simulink model "lateral_longiitude_distance"  (R2018a)
settings: Solver=FixedStepDiscrete  StartTime=0.0  StopTime=10.0  FixedStep=1  RelTol=1e-3
undefined symbols (not defined in the file or in its folder): BRAKING_ON_OFF, MUST_REQ
libraries: simulink x27
settings Model: Creator=S M Engineers  LastModifiedBy=S M Engineers

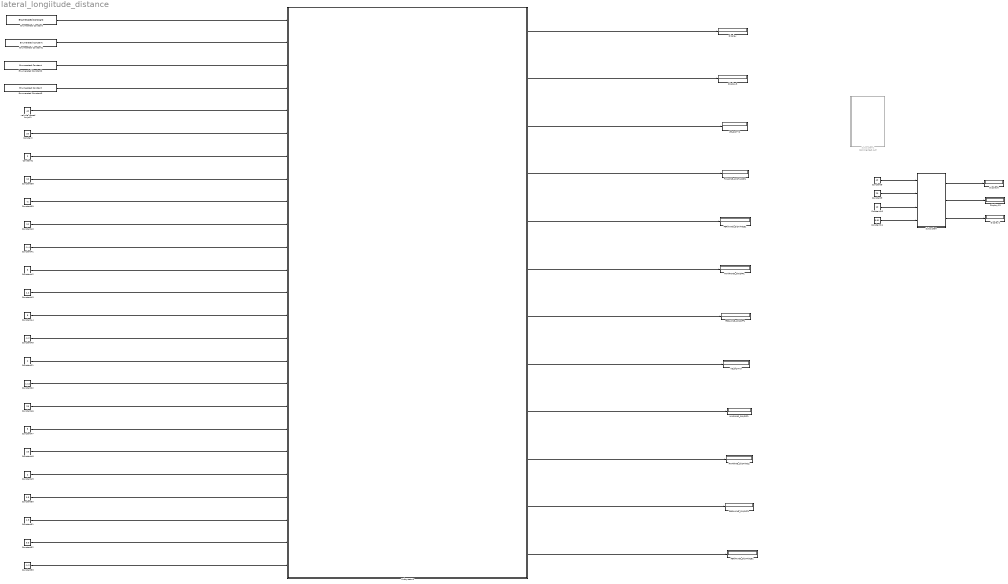
== system lateral_longiitude_distance ==
  Constant : Constant  Value=20
  Constant1 : Constant  Value=2
  Constant10 : Constant  Value=10
  Constant11 : Constant  Value=9.81
  Constant21 : Constant  Value=2
  Constant22 : Constant  Value=1.12
  Constant38 : Constant  Value=10
  Constant39 : Constant  Value=-2
  Constant40 : Constant  Value=12
  Constant41 : Constant  Value=-1.4
  Constant42 : Constant  Value=5
  Constant43 : Constant  Value=1.2
  Constant44 : Constant  Value=8
  Constant45 : Constant  Value=-1.2
  Constant46 : Constant  Value=25
  Constant47 : Constant  Value=5
  Constant48 : Constant  Value=16
  Constant49 : Constant  Value=2
  Constant50 : Constant  Value=0.5
  Constant51 : Constant  Value=1.3
  Constant52 : Constant  Value=0.3
  Constant53 : Constant  Value=-1.2
  Constant8 : Constant  Value=40
  Constant9 : Constant  Value=20
  Display{,2..3,6,13} (5 alike) : Display
  Enumerated Constant : simulink/Sources/Enumerated Constant  OutDataTypeStr=Enum: MUST_REQ  Value=MUST_REQ.IGNITION_ON  SampleTime=inf
      settings: SourceProductName=Simulink
  Enumerated Constant1 : simulink/Sources/Enumerated Constant  OutDataTypeStr=Enum: MUST_REQ  Value=MUST_REQ.EMERGENCY_BRAKING_ON  SampleTime=inf
      settings: SourceProductName=Simulink
  Enumerated Constant2 : simulink/Sources/Enumerated Constant  OutDataTypeStr=Enum: MUST_REQ  Value=MUST_REQ.DRIVE_MODE_ON  SampleTime=inf
      settings: SourceProductName=Simulink
  Enumerated Constant3 : simulink/Sources/Enumerated Constant  OutDataTypeStr=Enum: MUST_REQ  Value=MUST_REQ.REAR_MODE_OFF  SampleTime=inf
      settings: SourceProductName=Simulink
  FBRAIKNG_ON/OFF1 : Display
  FBRAKING_DISTANCE1 : Display
  FWARING_DISTANCE1 : Display
  FWARNING_ON/OFF1 : Display
  RBRAIKNG_ON/OFF1 : Display
  RBRAKING_DISTANCE1 : Display
  RWARING_DISTANC2 : Display
  Subsystem : Subsystem
  Subsystem1 : Subsystem  Commented=on
  Subsystem3 : Subsystem
      mask Display: image('Autonomous-Emergency-Braking-System-Market.jpg');
  VELOCITY2 : Display
  VELOCITY3 : Display
  WARNING_ON/OFF1 : Display
  vehicle speed km/ph1 : Constant  Value=40
  wires:
  Constant8/1 -> Subsystem/1(In1)
  Constant9/1 -> Subsystem/2(In2)
  Constant10/1 -> Subsystem/3(In3)
  Constant11/1 -> Subsystem/4(In4)
  Subsystem/1(Out1) -> Display6/1
  Subsystem/2(Out2) -> Display13/1
  Subsystem/3(Out3) -> Display2/1
  Enumerated Constant/1 -> Subsystem3/1(In1)
  Enumerated Constant1/1 -> Subsystem3/2(In2)
  Enumerated Constant2/1 -> Subsystem3/3(In3)
  Enumerated Constant3/1 -> Subsystem3/4(In4)
  vehicle speed km/ph1/1 -> Subsystem3/5(In5)
  Constant/1 -> Subsystem3/6(In6)
  Constant1/1 -> Subsystem3/7(In7)
  Constant38/1 -> Subsystem3/8(In8)
  Constant39/1 -> Subsystem3/9(In9)
  Constant40/1 -> Subsystem3/10(In10)
  Constant41/1 -> Subsystem3/11(In11)
  Constant42/1 -> Subsystem3/12(In12)
  Constant43/1 -> Subsystem3/13(In13)
  Constant44/1 -> Subsystem3/14(In14)
  Constant45/1 -> Subsystem3/15(In15)
  Constant21/1 -> Subsystem3/16(In16)
  Constant22/1 -> Subsystem3/17(In17)
  Constant46/1 -> Subsystem3/18(In18)
  Constant47/1 -> Subsystem3/19(In19)
  Constant48/1 -> Subsystem3/20(In20)
  Constant49/1 -> Subsystem3/21(In21)
  Constant50/1 -> Subsystem3/22(In22)
  Constant51/1 -> Subsystem3/23(In23)
  Constant52/1 -> Subsystem3/24(In24)
  Constant53/1 -> Subsystem3/25(In25)
  Subsystem3/1(Out1) -> Display/1
  Subsystem3/2(Out2) -> Display3/1
  Subsystem3/3(Out3) -> VELOCITY2/1
  Subsystem3/4(Out4) -> FWARING_DISTANCE1/1
  Subsystem3/5(Out5) -> FBRAKING_DISTANCE1/1
  Subsystem3/6(Out6) -> FWARNING_ON/OFF1/1
  Subsystem3/7(Out7) -> FBRAIKNG_ON/OFF1/1
  Subsystem3/8(Out8) -> VELOCITY3/1
  Subsystem3/9(Out9) -> WARNING_ON/OFF1/1
  Subsystem3/10(Out10) -> RWARING_DISTANC2/1
  Subsystem3/11(Out11) -> RBRAIKNG_ON/OFF1/1
  Subsystem3/12(Out12) -> RBRAKING_DISTANCE1/1

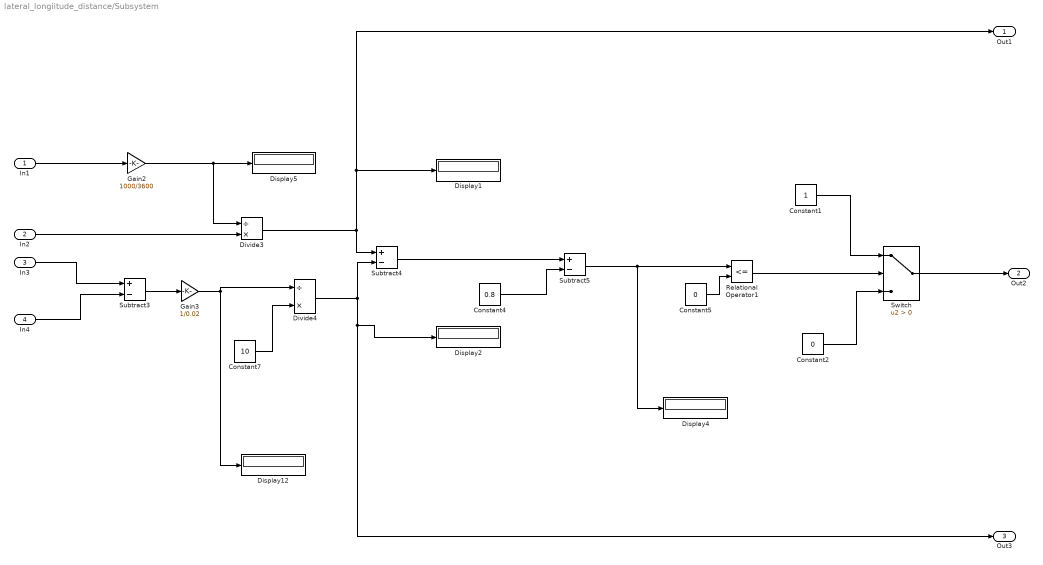
== system lateral_longiitude_distance/Subsystem ==
  In1 : Inport
  In2 : Inport  Port=2
  In3 : Inport  Port=3
  In4 : Inport  Port=4
  Constant1 : Constant
  Constant2 : Constant  Value=0
  Constant4 : Constant  Value=0.8
  Constant5 : Constant  Value=0
  Constant7 : Constant  Value=10
  Display{1..2,4..5,12} (5 alike) : Display
  Divide3 : Product  Inputs=/*
  Divide4 : Product  Inputs=/*
  Gain2 : Gain  Gain=1000/3600
  Gain3 : Gain  Gain=1/0.02
  Relational Operator1 : RelationalOperator  Operator=<=  OutDataTypeStr=boolean  RndMeth=Simplest
  Subtract3 : Sum  Inputs=+-
  Subtract4 : Sum  Inputs=+-
  Subtract5 : Sum  Inputs=+-
  Switch : Switch  Criteria=u2 > Threshold
  Out1 : Outport
  Out2 : Outport  Port=2
  Out3 : Outport  Port=3
  wires:
  In2/1 -> Divide3/2
  Constant4/1 -> Subtract5/2
  In1/1 -> Gain2/1
  Divide4/1 -> Display2/1, Out3/1, Subtract4/2
  Subtract3/1 -> Gain3/1
  Gain2/1 -> Divide3/1, Display5/1
  Gain3/1 -> Display12/1, Divide4/1
  Constant5/1 -> Relational Operator1/2
  In4/1 -> Subtract3/2
  Subtract5/1 -> Display4/1, Relational Operator1/1
  Constant7/1 -> Divide4/2
  Subtract4/1 -> Subtract5/1
  In3/1 -> Subtract3/1
  Divide3/1 -> Display1/1, Out1/1, Subtract4/1
  Switch/1 -> Out2/1
  Relational Operator1/1 -> Switch/2
  Constant1/1 -> Switch/1
  Constant2/1 -> Switch/3

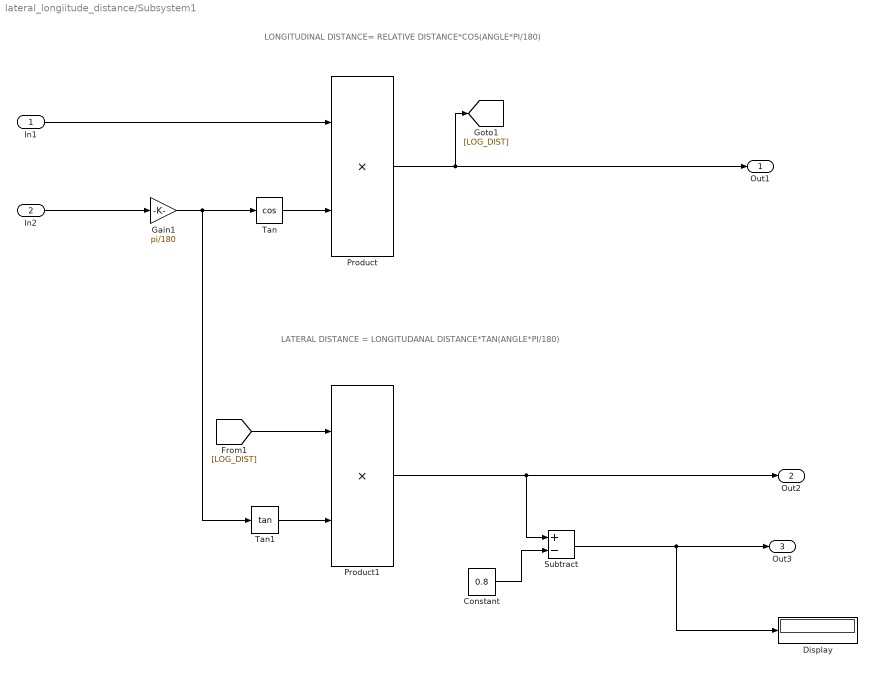
== system lateral_longiitude_distance/Subsystem1 ==
  note: LONGITUDINAL DISTANCE= RELATIVE DISTANCE*COS(ANGLE*PI/180)
  note: LATERAL DISTANCE = LONGITUDANAL DISTANCE*TAN(ANGLE*PI/180)
  In1 : Inport
  In2 : Inport  Port=2
  Constant : Constant  Value=0.8
  Display : Display
  Gain1 : Gain  Gain=pi/180
  Product : Product
  Product1 : Product
  Subtract : Sum  Inputs=+-
  Tan : Trigonometry  Operator=cos
  Tan1 : Trigonometry  Operator=tan
  Out1 : Outport
  Out2 : Outport  Port=2
  Out3 : Outport  Port=3
  wires:
  Gain1/1 -> Tan/1, Tan1/1
  Product1/1 -> Subtract/1, Out2/1
  Tan/1 -> Product/2
  [LOG_DIST] -> Product1/1
  Product/1 -> Out1/1, [LOG_DIST]
  In1/1 -> Product/1
  In2/1 -> Gain1/1
  Tan1/1 -> Product1/2
  Constant/1 -> Subtract/2
  Subtract/1 -> Out3/1, Display/1

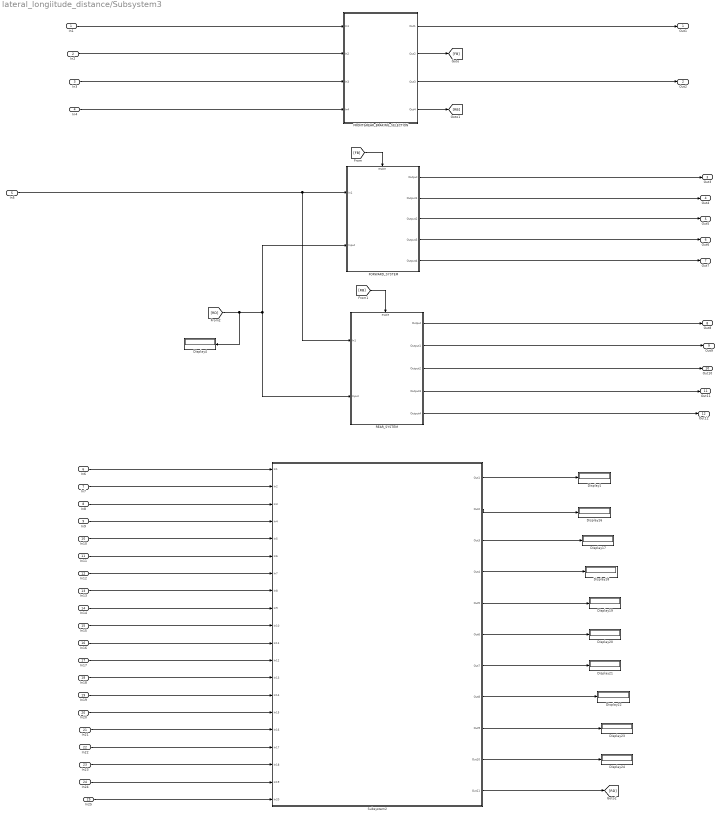
== system lateral_longiitude_distance/Subsystem3 ==
  In1 : Inport
  In2 : Inport  Port=2
  In3 : Inport  Port=3
  In4 : Inport  Port=4
  In5 : Inport  Port=5
  In6 : Inport  Port=6
  In7 : Inport  Port=7
  In8 : Inport  Port=8
  In9 : Inport  Port=9
  In10 : Inport  Port=10
  In11 : Inport  Port=11
  In12 : Inport  Port=12
  In13 : Inport  Port=13
  In14 : Inport  Port=14
  In15 : Inport  Port=15
  In16 : Inport  Port=16
  In17 : Inport  Port=17
  In18 : Inport  Port=18
  In19 : Inport  Port=19
  In20 : Inport  Port=20
  In21 : Inport  Port=21
  In22 : Inport  Port=22
  In23 : Inport  Port=23
  In24 : Inport  Port=24
  In25 : Inport  Port=25
  Display{1,4,16..24} (11 alike) : Display
  FORWARD_SYSTEM : Subsystem
  FRONT&REAR_BRAKING_SELECTION : Subsystem
  REAR_SYSTEM : Subsystem
  Subsystem2 : Subsystem
  Out1 : Outport
  Out2 : Outport  Port=2
  Out3 : Outport  Port=3
  Out4 : Outport  Port=4
  Out5 : Outport  Port=5
  Out6 : Outport  Port=6
  Out7 : Outport  Port=7
  Out8 : Outport  Port=8
  Out9 : Outport  Port=9
  Out10 : Outport  Port=10
  Out11 : Outport  Port=11
  Out12 : Outport  Port=12
  wires:
  FORWARD_SYSTEM/5(Output4) -> Out7/1
  In17/1 -> Subsystem2/12(In12)
  In23/1 -> Subsystem2/18(In18)
  [RD] -> Display4/1, REAR_SYSTEM/2(Input), FORWARD_SYSTEM/2(Input)
  In12/1 -> Subsystem2/7(In7)
  In5/1 -> REAR_SYSTEM/1(In1), FORWARD_SYSTEM/1(In1)
  FRONT&REAR_BRAKING_SELECTION/4(Out4) -> [RB]
  FRONT&REAR_BRAKING_SELECTION/1(Out1) -> Out1/1
  In20/1 -> Subsystem2/15(In15)
  Subsystem2/5(Out5) -> Display19/1
  Subsystem2/4(Out4) -> Display18/1
  In10/1 -> Subsystem2/5(In5)
  Subsystem2/10(Out10) -> Display24/1
  REAR_SYSTEM/5(Output4) -> Out12/1
  Subsystem2/3(Out3) -> Display17/1
  Subsystem2/9(Out9) -> Display23/1
  In8/1 -> Subsystem2/3(In3)
  Subsystem2/1(Out1) -> Display1/1
  REAR_SYSTEM/4(Output3) -> Out11/1
  Subsystem2/2(Out2) -> Display16/1
  In2/1 -> FRONT&REAR_BRAKING_SELECTION/2(In2)
  In6/1 -> Subsystem2/1(In1)
  FRONT&REAR_BRAKING_SELECTION/3(Out3) -> Out2/1
  In15/1 -> Subsystem2/10(In10)
  REAR_SYSTEM/2(Output1) -> Out9/1
  [RB] -> REAR_SYSTEM/Enable
  In16/1 -> Subsystem2/11(In11)
  Subsystem2/7(Out7) -> Display21/1
  Subsystem2/6(Out6) -> Display20/1
  FORWARD_SYSTEM/4(Output3) -> Out6/1
  Subsystem2/8(Out8) -> Display22/1
  In1/1 -> FRONT&REAR_BRAKING_SELECTION/1(In1)
  In13/1 -> Subsystem2/8(In8)
  Subsystem2/11(Out11) -> [RD]
  In24/1 -> Subsystem2/19(In19)
  FRONT&REAR_BRAKING_SELECTION/2(Out2) -> [FB]
  In14/1 -> Subsystem2/9(In9)
  In22/1 -> Subsystem2/17(In17)
  [FB] -> FORWARD_SYSTEM/Enable
  In11/1 -> Subsystem2/6(In6)
  FORWARD_SYSTEM/1(Output) -> Out3/1
  In25/1 -> Subsystem2/20(In20)
  REAR_SYSTEM/1(Output) -> Out8/1
  In9/1 -> Subsystem2/4(In4)
  In7/1 -> Subsystem2/2(In2)
  In21/1 -> Subsystem2/16(In16)
  In19/1 -> Subsystem2/14(In14)
  In18/1 -> Subsystem2/13(In13)
  FORWARD_SYSTEM/2(Output1) -> Out4/1
  In4/1 -> FRONT&REAR_BRAKING_SELECTION/4(In4)
  REAR_SYSTEM/3(Output2) -> Out10/1
  In3/1 -> FRONT&REAR_BRAKING_SELECTION/3(In3)
  FORWARD_SYSTEM/3(Output2) -> Out5/1

== system lateral_longiitude_distance/Subsystem3/FORWARD_SYSTEM ==
  In1 : Inport
  Input : Inport  Port=2
  Enable : EnablePort
  "FORWARD_EMERGENCY_BRAKING_SYSTEM " : Subsystem
  Output : Outport
  Output1 : Outport  Port=2
  Output2 : Outport  Port=3
  Output3 : Outport  Port=4
  Output4 : Outport  Port=5
  wires:
  In1/1 -> "FORWARD_EMERGENCY_BRAKING_SYSTEM "/1(In1)
  Input/1 -> "FORWARD_EMERGENCY_BRAKING_SYSTEM "/2(Input)
  "FORWARD_EMERGENCY_BRAKING_SYSTEM "/1(Out5) -> Output/1  "VELOCITY M/S"
  "FORWARD_EMERGENCY_BRAKING_SYSTEM "/2(Out1) -> Output1/1  "WARNING DISTANCE"
  "FORWARD_EMERGENCY_BRAKING_SYSTEM "/3(Out2) -> Output2/1  "BRAKING DISTANCE"
  "FORWARD_EMERGENCY_BRAKING_SYSTEM "/4(Out3) -> Output3/1  "WARNING"
  "FORWARD_EMERGENCY_BRAKING_SYSTEM "/5(Out4) -> Output4/1  "BRAKING"

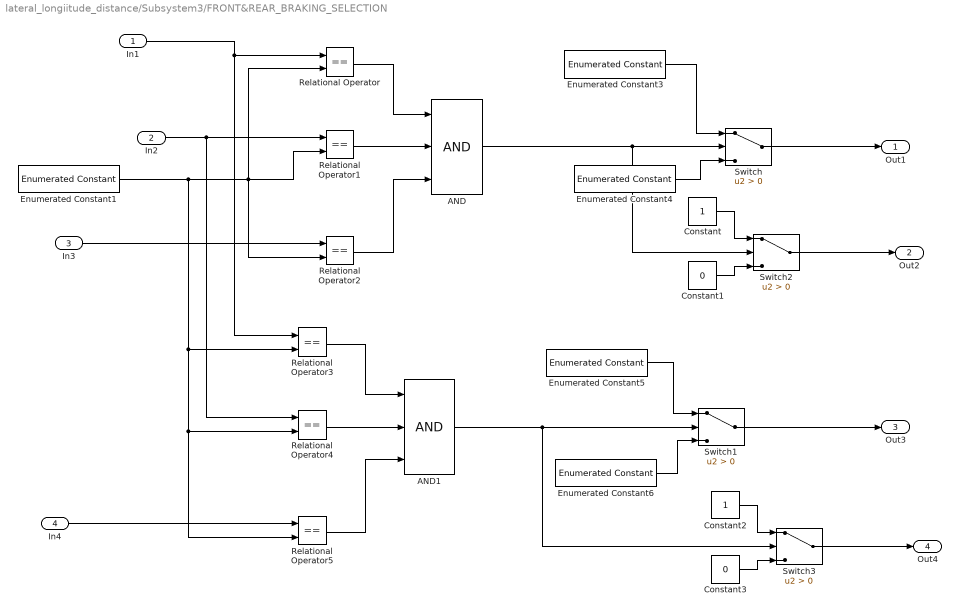
== system lateral_longiitude_distance/Subsystem3/FRONT&REAR_BRAKING_SELECTION ==
  In1 : Inport
  In2 : Inport  Port=2
  In3 : Inport  Port=3
  In4 : Inport  Port=4
  AND : Logic  Inputs=3  AllPortsSameDT=off  OutDataTypeStr=boolean
  AND1 : Logic  Inputs=3  AllPortsSameDT=off  OutDataTypeStr=boolean
  Constant : Constant
  Constant1 : Constant  Value=0
  Constant2 : Constant
  Constant3 : Constant  Value=0
  Enumerated Constant1 : simulink/Sources/Enumerated Constant  OutDataTypeStr=Enum: MUST_REQ  Value=MUST_REQ.COMPARE_WITH_ALL  SampleTime=inf
      settings: SourceProductName=Simulink
  Enumerated Constant3 : simulink/Sources/Enumerated Constant  OutDataTypeStr=Enum: BRAKING_ON_OFF  Value=BRAKING_ON_OFF.FRONT_BRAKING_ON  SampleTime=inf
      settings: SourceProductName=Simulink
  Enumerated Constant4 : simulink/Sources/Enumerated Constant  OutDataTypeStr=Enum: BRAKING_ON_OFF  Value=BRAKING_ON_OFF.NONE  SampleTime=inf
      settings: SourceProductName=Simulink
  Enumerated Constant5 : simulink/Sources/Enumerated Constant  OutDataTypeStr=Enum: BRAKING_ON_OFF  Value=BRAKING_ON_OFF.REAR_BRAKING_ON  SampleTime=inf
      settings: SourceProductName=Simulink
  Enumerated Constant6 : simulink/Sources/Enumerated Constant  OutDataTypeStr=Enum: BRAKING_ON_OFF  Value=BRAKING_ON_OFF.NONE  SampleTime=inf
      settings: SourceProductName=Simulink
  Relational Operator{,1..5} (6 alike) : RelationalOperator  Operator===  OutDataTypeStr=boolean  RndMeth=Simplest
  Switch{,1..3} (4 alike) : Switch  Criteria=u2 > Threshold
  Out1 : Outport
  Out2 : Outport  Port=2
  Out3 : Outport  Port=3
  Out4 : Outport  Port=4
  wires:
  Relational Operator/1 -> AND/1
  Relational Operator1/1 -> AND/2
  Relational Operator2/1 -> AND/3
  AND/1 -> Switch2/2, Switch/2
  Switch/1 -> Out1/1
  Enumerated Constant3/1 -> Switch/1
  Enumerated Constant4/1 -> Switch/3
  Switch1/1 -> Out3/1
  Enumerated Constant5/1 -> Switch1/1
  Enumerated Constant6/1 -> Switch1/3
  Enumerated Constant1/1 -> Relational Operator4/2, Relational Operator5/2, Relational Operator3/2, Relational Operator2/2, Relational Operator/2, Relational Operator1/2
  In2/1 -> Relational Operator4/1, Relational Operator1/1
  Relational Operator5/1 -> AND1/3
  Relational Operator4/1 -> AND1/2
  In1/1 -> Relational Operator3/1, Relational Operator/1
  Relational Operator3/1 -> AND1/1
  In4/1 -> Relational Operator5/1
  In3/1 -> Relational Operator2/1
  Constant/1 -> Switch2/1
  Constant1/1 -> Switch2/3
  Switch2/1 -> Out2/1
  Switch3/1 -> Out4/1
  Constant3/1 -> Switch3/3
  Constant2/1 -> Switch3/1
  AND1/1 -> Switch1/2, Switch3/2

== system lateral_longiitude_distance/Subsystem3/REAR_SYSTEM ==
  In1 : Inport
  Input : Inport  Port=2
  Enable : EnablePort
  "REAR_EMERGENCY_BRAKING_SYSTEM " : Subsystem
  Output : Outport
  Output1 : Outport  Port=2
  Output2 : Outport  Port=3
  Output3 : Outport  Port=4
  Output4 : Outport  Port=5
  wires:
  "REAR_EMERGENCY_BRAKING_SYSTEM "/5(Out4) -> Output4/1  "BRAKING"
  "REAR_EMERGENCY_BRAKING_SYSTEM "/4(Out3) -> Output3/1  "WARNING"
  "REAR_EMERGENCY_BRAKING_SYSTEM "/3(Out2) -> Output2/1  "BRAKING DISTANCE"
  "REAR_EMERGENCY_BRAKING_SYSTEM "/2(Out1) -> Output1/1  "WARNING DISTANCE"
  "REAR_EMERGENCY_BRAKING_SYSTEM "/1(Out5) -> Output/1  "VELOCITY M/S"
  Input/1 -> "REAR_EMERGENCY_BRAKING_SYSTEM "/2(Input)
  In1/1 -> "REAR_EMERGENCY_BRAKING_SYSTEM "/1(In1)

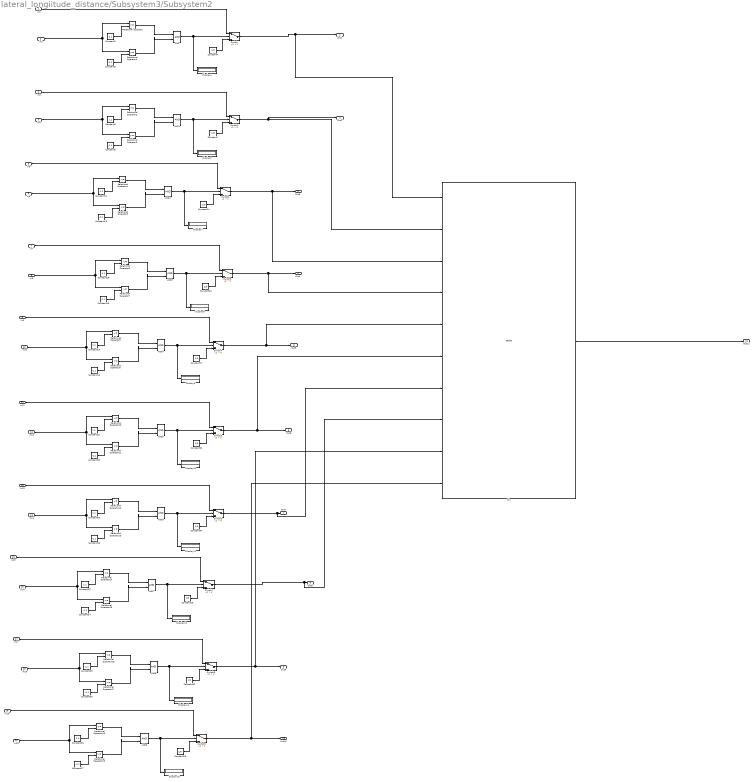
== system lateral_longiitude_distance/Subsystem3/Subsystem2 ==
  In1 : Inport
  In2 : Inport  Port=2
  In3 : Inport  Port=3
  In4 : Inport  Port=4
  In5 : Inport  Port=5
  In6 : Inport  Port=6
  In7 : Inport  Port=7
  In8 : Inport  Port=8
  In9 : Inport  Port=9
  In10 : Inport  Port=10
  In11 : Inport  Port=11
  In12 : Inport  Port=12
  In13 : Inport  Port=13
  In14 : Inport  Port=14
  In15 : Inport  Port=15
  In16 : Inport  Port=16
  In17 : Inport  Port=17
  In18 : Inport  Port=18
  In19 : Inport  Port=19
  In20 : Inport  Port=20
  AND{,1..9} (10 alike) : Logic  IconShape=distinctive  AllPortsSameDT=off  OutDataTypeStr=boolean
  Constant{2,5,12,15,18,23,26,29,31,35} (10 alike) : Constant  Value=1.1
  Constant{3,6,13,16,19,24,27,30,33,36} (10 alike) : Constant  Value=-1.1
  Constant{4,7,14,17,20,25,28,32,34,37} (10 alike) : Constant  Value=1/0
  Display{4..5,7..12,14..15} (10 alike) : Display
  Min : MinMax  Inputs=10
  Relational Operator{,2,4,6,8,10,12,14,16,18} (10 alike) : RelationalOperator  Operator=<=  OutDataTypeStr=boolean  RndMeth=Simplest
  Relational Operator{1,3,5,7,9,11,13,15,17,19} (10 alike) : RelationalOperator  OutDataTypeStr=boolean  RndMeth=Simplest
  Switch{,1..9} (10 alike) : Switch  Criteria=u2 > Threshold
  Out1 : Outport
  Out2 : Outport  Port=2
  Out3 : Outport  Port=3
  Out4 : Outport  Port=4
  Out5 : Outport  Port=5
  Out6 : Outport  Port=6
  Out7 : Outport  Port=7
  Out8 : Outport  Port=8
  Out9 : Outport  Port=9
  Out10 : Outport  Port=10
  Out11 : Outport  Port=11
  wires:
  Constant17/1 -> Switch4/3
  Relational Operator2/1 -> AND1/1
  In3/1 -> Switch1/1
  AND5/1 -> Switch5/2, Display10/1
  In16/1 -> Relational Operator15/1, Relational Operator14/1
  In4/1 -> Relational Operator3/1, Relational Operator2/1
  AND2/1 -> Display7/1, Switch2/2
  Constant24/1 -> Relational Operator15/2
  AND1/1 -> Switch1/2, Display5/1
  Relational Operator12/1 -> AND6/1
  Constant35/1 -> Relational Operator12/2
  Constant37/1 -> Switch6/3
  Constant34/1 -> Switch5/3
  Relational Operator13/1 -> AND6/2
  Relational Operator7/1 -> AND3/2
  Relational Operator10/1 -> AND5/1
  Relational Operator11/1 -> AND5/2
  In12/1 -> Relational Operator11/1, Relational Operator10/1
  AND8/1 -> Switch8/2, Display14/1
  In13/1 -> Switch6/1
  Constant31/1 -> Relational Operator10/2
  AND6/1 -> Display11/1, Switch6/2
  AND9/1 -> Display15/1, Switch9/2
  Switch6/1 -> Min/7, Out7/1
  Constant33/1 -> Relational Operator11/2
  AND3/1 -> Display8/1, Switch3/2
  Constant3/1 -> Relational Operator1/2
  AND4/1 -> Switch4/2, Display9/1
  In20/1 -> Relational Operator18/1, Relational Operator19/1
  Constant30/1 -> Relational Operator17/2
  Constant6/1 -> Relational Operator3/2
  Constant32/1 -> Switch8/3
  Constant27/1 -> Relational Operator19/2
  Constant29/1 -> Relational Operator16/2
  Constant26/1 -> Relational Operator18/2
  Relational Operator18/1 -> AND9/1
  Relational Operator1/1 -> AND/2
  Switch5/1 -> Min/6, Out6/1
  Relational Operator17/1 -> AND8/2
  In18/1 -> Relational Operator17/1, Relational Operator16/1
  Relational Operator16/1 -> AND8/1
  Constant20/1 -> Switch3/3
  Constant25/1 -> Switch7/3
  Relational Operator14/1 -> AND7/1
  Switch3/1 -> Min/4, Out4/1
  Constant16/1 -> Relational Operator9/2
  In10/1 -> Relational Operator9/1, Relational Operator8/1
  Relational Operator19/1 -> AND9/2
  Constant5/1 -> Relational Operator2/2
  Constant7/1 -> Switch1/3
  Constant28/1 -> Switch9/3
  Constant23/1 -> Relational Operator14/2
  Constant19/1 -> Relational Operator7/2
  In5/1 -> Switch2/1
  In8/1 -> Relational Operator6/1, Relational Operator7/1
  Relational Operator15/1 -> AND7/2
  In14/1 -> Relational Operator12/1, Relational Operator13/1
  Constant36/1 -> Relational Operator13/2
  AND7/1 -> Switch7/2, Display12/1
  Switch/1 -> Min/1, Out1/1
  Constant13/1 -> Relational Operator5/2
  AND/1 -> Display4/1, Switch/2
  Relational Operator3/1 -> AND1/2
  Constant15/1 -> Relational Operator8/2
  Constant18/1 -> Relational Operator6/2
  Relational Operator6/1 -> AND3/1
  Relational Operator/1 -> AND/1
  Constant4/1 -> Switch/3
  In2/1 -> Relational Operator/1, Relational Operator1/1
  Constant2/1 -> Relational Operator/2
  In6/1 -> Relational Operator4/1, Relational Operator5/1
  Constant12/1 -> Relational Operator4/2
  Relational Operator8/1 -> AND4/1
  Relational Operator9/1 -> AND4/2
  Constant14/1 -> Switch2/3
  Relational Operator5/1 -> AND2/2
  Relational Operator4/1 -> AND2/1
  In19/1 -> Switch9/1
  In11/1 -> Switch5/1
  In17/1 -> Switch8/1
  Switch1/1 -> Min/2, Out2/1
  Switch2/1 -> Min/3, Out3/1
  Switch8/1 -> Min/9, Out9/1
  Switch9/1 -> Min/10, Out10/1
  In9/1 -> Switch4/1
  In1/1 -> Switch/1
  Switch4/1 -> Min/5, Out5/1
  In7/1 -> Switch3/1
  In15/1 -> Switch7/1
  Switch7/1 -> Min/8, Out8/1
  Min/1 -> Out11/1

== system lateral_longiitude_distance/Subsystem3/FORWARD_SYSTEM/FORWARD_EMERGENCY_BRAKING_SYSTEM  ==
  In1 : Inport
  Input : Inport  Port=2
  GREATER_THAN_60 : Subsystem
  Gain : Gain  Gain=1000/3600
  LESS_THAN_60 : Subsystem
  Subsystem1 : Subsystem
  comp_To_60 : Subsystem
  Out5 : Outport
  Out1 : Outport  Port=2
  Out2 : Outport  Port=3
  Out3 : Outport  Port=4
  Out4 : Outport  Port=5
  wires:
  In1/1 -> Gain/1
  comp_To_60/1(Out1) -> LESS_THAN_60/Enable
  comp_To_60/2(Out2) -> GREATER_THAN_60/Enable
  Input/1 -> GREATER_THAN_60/2(Input), LESS_THAN_60/2(Input)
  Gain/1 -> Out5/1, GREATER_THAN_60/1(In1), LESS_THAN_60/1(In1), comp_To_60/1(In1)  "VELOCITY M/S"
  LESS_THAN_60/1(Output) -> Subsystem1/1(In1)
  LESS_THAN_60/2(Out2) -> Subsystem1/2(In2)
  LESS_THAN_60/3(Out3) -> Subsystem1/3(In3)
  LESS_THAN_60/4(Output1) -> Subsystem1/4(In4)
  GREATER_THAN_60/1(Output) -> Subsystem1/5(In5)
  GREATER_THAN_60/2(Output1) -> Subsystem1/6(In6)
  GREATER_THAN_60/3(Output2) -> Subsystem1/7(In7)
  GREATER_THAN_60/4(Output3) -> Subsystem1/8(In8)
  Subsystem1/1(Out1) -> Out1/1  "WARNING DISTANCE"
  Subsystem1/2(Out2) -> Out2/1  "BRAKING DISTANCE"
  Subsystem1/3(Out3) -> Out3/1  "WARNING"
  Subsystem1/4(Out4) -> Out4/1  "BRAKING"

== system lateral_longiitude_distance/Subsystem3/REAR_SYSTEM/REAR_EMERGENCY_BRAKING_SYSTEM  ==
  In1 : Inport
  Input : Inport  Port=2
  GREATER_THAN_40 : Subsystem
  Gain : Gain  Gain=1000/3600
  LESS_THAN_40 : Subsystem
  Subsystem1 : Subsystem
  comp_To_40 : Subsystem
  Out5 : Outport
  Out1 : Outport  Port=2
  Out2 : Outport  Port=3
  Out3 : Outport  Port=4
  Out4 : Outport  Port=5
  wires:
  Subsystem1/4(Out4) -> Out4/1  "BRAKING"
  Subsystem1/3(Out3) -> Out3/1  "WARNING"
  Subsystem1/2(Out2) -> Out2/1  "BRAKING DISTANCE"
  Subsystem1/1(Out1) -> Out1/1  "WARNING DISTANCE"
  GREATER_THAN_40/4(Output3) -> Subsystem1/8(In8)
  GREATER_THAN_40/3(Output2) -> Subsystem1/7(In7)
  GREATER_THAN_40/2(Output1) -> Subsystem1/6(In6)
  GREATER_THAN_40/1(Output) -> Subsystem1/5(In5)
  LESS_THAN_40/4(Output1) -> Subsystem1/4(In4)
  LESS_THAN_40/3(Out3) -> Subsystem1/3(In3)
  LESS_THAN_40/2(Out2) -> Subsystem1/2(In2)
  LESS_THAN_40/1(Output) -> Subsystem1/1(In1)
  Gain/1 -> comp_To_40/1(In1), LESS_THAN_40/1(In1), GREATER_THAN_40/1(In1), Out5/1  "VELOCITY M/S"
  Input/1 -> LESS_THAN_40/2(Input), GREATER_THAN_40/2(Input)
  comp_To_40/2(Out2) -> GREATER_THAN_40/Enable
  comp_To_40/1(Out1) -> LESS_THAN_40/Enable
  In1/1 -> Gain/1

== system lateral_longiitude_distance/Subsystem3/FORWARD_SYSTEM/FORWARD_EMERGENCY_BRAKING_SYSTEM /GREATER_THAN_60 ==
  In1 : Inport
  Input : Inport  Port=2
  Enable : EnablePort
  B_D : Subsystem
  W_D : Subsystem
  Output : Outport
  Output1 : Outport  Port=2
  Output2 : Outport  Port=3
  Output3 : Outport  Port=4
  wires:
  W_D/1(Output) -> Output/1
  W_D/2(Output1) -> Output1/1
  B_D/1(Output) -> Output2/1
  B_D/2(Output1) -> Output3/1
  Input/1 -> W_D/2(Input), B_D/2(Input)
  In1/1 -> B_D/1(In1), W_D/1(In1)

== system lateral_longiitude_distance/Subsystem3/FORWARD_SYSTEM/FORWARD_EMERGENCY_BRAKING_SYSTEM /LESS_THAN_60 ==
  In1 : Inport
  Input : Inport  Port=2
  Enable : EnablePort
  B_D : Subsystem
  Spd_Km_m1 : Subsystem  Commented=on
  W_D : Subsystem
  Output : Outport
  Out2 : Outport  Port=2
  Out3 : Outport  Port=3
  Output1 : Outport  Port=4
  wires:
  In1/1 -> B_D/1(In1), W_D/1(In1)
  Input/1 -> W_D/2(Input), B_D/2(Input)
  W_D/1(Output) -> Output/1
  W_D/2(Output1) -> Out2/1
  B_D/1(Output) -> Out3/1
  B_D/2(Output1) -> Output1/1

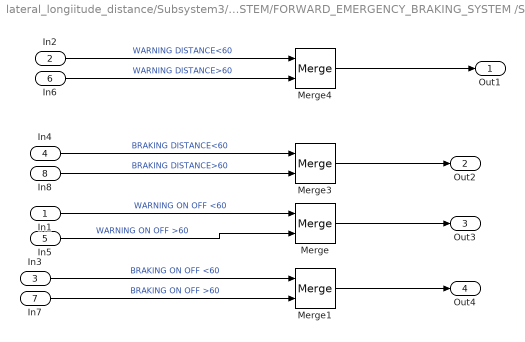
== system lateral_longiitude_distance/Subsystem3/FORWARD_SYSTEM/FORWARD_EMERGENCY_BRAKING_SYSTEM /Subsystem1 ==
  In1 : Inport
  In2 : Inport  Port=2
  In3 : Inport  Port=3
  In4 : Inport  Port=4
  In5 : Inport  Port=5
  In6 : Inport  Port=6
  In7 : Inport  Port=7
  In8 : Inport  Port=8
  Merge{,1,3..4} (4 alike) : Merge
  Out1 : Outport
  Out2 : Outport  Port=2
  Out3 : Outport  Port=3
  Out4 : Outport  Port=4
  wires:
  In2/1 -> Merge4/1  "WARNING DISTANCE<60"
  In7/1 -> Merge1/2  "BRAKING ON OFF >60"
  Merge4/1 -> Out1/1
  Merge/1 -> Out3/1
  In3/1 -> Merge1/1  "BRAKING ON OFF <60"
  In8/1 -> Merge3/2  "BRAKING DISTANCE>60"
  In4/1 -> Merge3/1  "BRAKING DISTANCE<60"
  In6/1 -> Merge4/2  "WARNING DISTANCE>60"
  In5/1 -> Merge/2  "WARNING ON OFF >60"
  Merge3/1 -> Out2/1
  In1/1 -> Merge/1  "WARNING ON OFF <60"
  Merge1/1 -> Out4/1

== system lateral_longiitude_distance/Subsystem3/FORWARD_SYSTEM/FORWARD_EMERGENCY_BRAKING_SYSTEM /comp_To_60 ==
  In1 : Inport
  Compare To Constant : simulink/Logic and Bit Operations/Compare To Constant  relop=>=  const=60  OutDataTypeStr=boolean
  NOT : Logic  Operator=NOT  IconShape=distinctive  AllPortsSameDT=off  OutDataTypeStr=boolean
  Out1 : Outport
  Out2 : Outport  Port=2
  wires:
  Compare To Constant/1 -> Out2/1, NOT/1
  NOT/1 -> Out1/1
  In1/1 -> Compare To Constant/1

== system lateral_longiitude_distance/Subsystem3/REAR_SYSTEM/REAR_EMERGENCY_BRAKING_SYSTEM /GREATER_THAN_40 ==
  In1 : Inport
  Input : Inport  Port=2
  Enable : EnablePort
  B_D : Subsystem
  W_D : Subsystem
  Output : Outport
  Output1 : Outport  Port=2
  Output2 : Outport  Port=3
  Output3 : Outport  Port=4
  wires:
  In1/1 -> W_D/1(In1), B_D/1(In1)
  Input/1 -> B_D/2(Input), W_D/2(Input)
  B_D/2(Output1) -> Output3/1
  B_D/1(Output) -> Output2/1
  W_D/2(Output1) -> Output1/1
  W_D/1(Output) -> Output/1

== system lateral_longiitude_distance/Subsystem3/REAR_SYSTEM/REAR_EMERGENCY_BRAKING_SYSTEM /LESS_THAN_40 ==
  In1 : Inport
  Input : Inport  Port=2
  Enable : EnablePort
  B_D : Subsystem
  W_D : Subsystem
  Output : Outport
  Out2 : Outport  Port=2
  Out3 : Outport  Port=3
  Output1 : Outport  Port=4
  wires:
  B_D/2(Output1) -> Output1/1
  B_D/1(Output) -> Out3/1
  W_D/2(Output1) -> Out2/1
  W_D/1(Output) -> Output/1
  Input/1 -> B_D/2(Input), W_D/2(Input)
  In1/1 -> B_D/1(In1), W_D/1(In1)

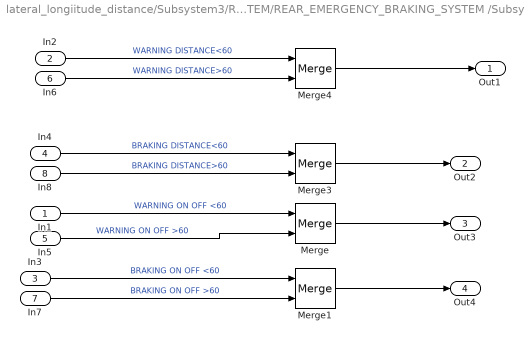
== system lateral_longiitude_distance/Subsystem3/REAR_SYSTEM/REAR_EMERGENCY_BRAKING_SYSTEM /Subsystem1 ==
  In1 : Inport
  In2 : Inport  Port=2
  In3 : Inport  Port=3
  In4 : Inport  Port=4
  In5 : Inport  Port=5
  In6 : Inport  Port=6
  In7 : Inport  Port=7
  In8 : Inport  Port=8
  Merge{,1,3..4} (4 alike) : Merge
  Out1 : Outport
  Out2 : Outport  Port=2
  Out3 : Outport  Port=3
  Out4 : Outport  Port=4
  wires:
  Merge1/1 -> Out4/1
  In1/1 -> Merge/1  "WARNING ON OFF <60"
  Merge3/1 -> Out2/1
  In5/1 -> Merge/2  "WARNING ON OFF >60"
  In6/1 -> Merge4/2  "WARNING DISTANCE>60"
  In4/1 -> Merge3/1  "BRAKING DISTANCE<60"
  In8/1 -> Merge3/2  "BRAKING DISTANCE>60"
  In3/1 -> Merge1/1  "BRAKING ON OFF <60"
  Merge/1 -> Out3/1
  Merge4/1 -> Out1/1
  In7/1 -> Merge1/2  "BRAKING ON OFF >60"
  In2/1 -> Merge4/1  "WARNING DISTANCE<60"

== system lateral_longiitude_distance/Subsystem3/REAR_SYSTEM/REAR_EMERGENCY_BRAKING_SYSTEM /comp_To_40 ==
  In1 : Inport
  Compare To Constant : simulink/Logic and Bit Operations/Compare To Constant  relop=>=  const=40  OutDataTypeStr=boolean
  NOT : Logic  Operator=NOT  IconShape=distinctive  AllPortsSameDT=off  OutDataTypeStr=boolean
  Out1 : Outport
  Out2 : Outport  Port=2
  wires:
  In1/1 -> Compare To Constant/1
  NOT/1 -> Out1/1
  Compare To Constant/1 -> NOT/1, Out2/1

== system lateral_longiitude_distance/Subsystem3/FORWARD_SYSTEM/FORWARD_EMERGENCY_BRAKING_SYSTEM /GREATER_THAN_60/B_D ==
  note: Braking Distance=((V1*V1)/(0.7*2*9.81))*1000
  In1 : Inport
  Input : Inport  Port=2
  Divide1 : Product  Inputs=*/
  Enumerated Constant : simulink/Sources/Enumerated Constant  OutDataTypeStr=Enum: BRAKING_ON_OFF  Value=BRAKING_ON_OFF.FRONT_WARNING_ON  SampleTime=inf
      settings: SourceProductName=Simulink
  Enumerated Constant1 : simulink/Sources/Enumerated Constant  OutDataTypeStr=Enum: BRAKING_ON_OFF  Value=BRAKING_ON_OFF.BRAKING_OFF  SampleTime=inf
      settings: SourceProductName=Simulink
  Fric : Constant  Value=0.7
  Product1 : Product  Inputs=3
  Relational Operator : RelationalOperator  Operator=<=  OutDataTypeStr=boolean  RndMeth=Simplest
  Square : Math  Operator=square  SaturateOnIntegerOverflow=on
  Switch : Switch  Criteria=u2 > Threshold
  constant : Constant  Value=2
  g : Constant  Value=9.81
  Output : Outport
  Output1 : Outport  Port=2
  wires:
  Square/1 -> Divide1/1
  In1/1 -> Square/1
  constant/1 -> Product1/2
  Fric/1 -> Product1/1
  Product1/1 -> Divide1/2
  g/1 -> Product1/3
  Switch/1 -> Output/1
  Enumerated Constant1/1 -> Switch/3
  Enumerated Constant/1 -> Switch/1
  Relational Operator/1 -> Switch/2
  Divide1/1 -> Relational Operator/2, Output1/1
  Input/1 -> Relational Operator/1

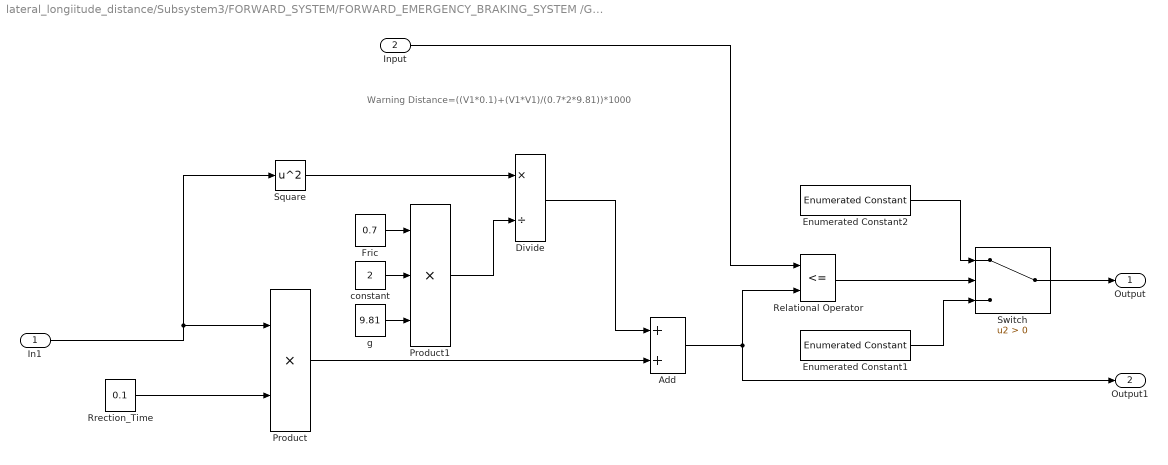
== system lateral_longiitude_distance/Subsystem3/FORWARD_SYSTEM/FORWARD_EMERGENCY_BRAKING_SYSTEM /GREATER_THAN_60/W_D ==
  note: Warning Distance=((V1*0.1)+(V1*V1)/(0.7*2*9.81))*1000
  In1 : Inport
  Input : Inport  Port=2
  Add : Sum
  Divide : Product  Inputs=*/
  Enumerated Constant1 : simulink/Sources/Enumerated Constant  OutDataTypeStr=Enum: BRAKING_ON_OFF  Value=BRAKING_ON_OFF.WARNING_OFF  SampleTime=inf
      settings: SourceProductName=Simulink
  Enumerated Constant2 : simulink/Sources/Enumerated Constant  OutDataTypeStr=Enum: BRAKING_ON_OFF  Value=BRAKING_ON_OFF.FRONT_WARNING_ON  SampleTime=inf
      settings: SourceProductName=Simulink
  Fric : Constant  Value=0.7
  Product : Product
  Product1 : Product  Inputs=3
  Relational Operator : RelationalOperator  Operator=<=  OutDataTypeStr=boolean  RndMeth=Simplest
  "Rrection_Time " : Constant  Value=0.1
  Square : Math  Operator=square  SaturateOnIntegerOverflow=on
  Switch : Switch  Criteria=u2 > Threshold
  constant : Constant  Value=2
  g : Constant  Value=9.81
  Output : Outport
  Output1 : Outport  Port=2
  wires:
  Product1/1 -> Divide/2
  Square/1 -> Divide/1
  Product/1 -> Add/2
  In1/1 -> Square/1, Product/1
  "Rrection_Time "/1 -> Product/2
  Divide/1 -> Add/1
  Fric/1 -> Product1/1
  constant/1 -> Product1/2
  g/1 -> Product1/3
  Switch/1 -> Output/1
  Enumerated Constant1/1 -> Switch/3
  Enumerated Constant2/1 -> Switch/1
  Relational Operator/1 -> Switch/2
  Add/1 -> Output1/1, Relational Operator/2
  Input/1 -> Relational Operator/1

== system lateral_longiitude_distance/Subsystem3/FORWARD_SYSTEM/FORWARD_EMERGENCY_BRAKING_SYSTEM /LESS_THAN_60/B_D ==
  note: Braking Distance=((V1*V1)/(1*2*9.81))
  In1 : Inport
  Input : Inport  Port=2
  Divide1 : Product  Inputs=*/
  Enumerated Constant : simulink/Sources/Enumerated Constant  OutDataTypeStr=Enum: BRAKING_ON_OFF  Value=BRAKING_ON_OFF.FRONT_BRAKING_ON  SampleTime=inf
      settings: SourceProductName=Simulink
  Enumerated Constant1 : simulink/Sources/Enumerated Constant  OutDataTypeStr=Enum: BRAKING_ON_OFF  Value=BRAKING_ON_OFF.BRAKING_OFF  SampleTime=inf
      settings: SourceProductName=Simulink
  Fric : Constant
  Product1 : Product  Inputs=3
  Relational Operator : RelationalOperator  Operator=<=  OutDataTypeStr=boolean  RndMeth=Simplest
  Square : Math  Operator=square  SaturateOnIntegerOverflow=on
  Switch : Switch  Criteria=u2 > Threshold
  constant : Constant  Value=2
  g : Constant  Value=9.81
  Output : Outport
  Output1 : Outport  Port=2
  wires:
  In1/1 -> Square/1
  Square/1 -> Divide1/1
  constant/1 -> Product1/1
  Fric/1 -> Product1/2
  g/1 -> Product1/3
  Product1/1 -> Divide1/2
  Switch/1 -> Output/1
  Enumerated Constant1/1 -> Switch/3
  Enumerated Constant/1 -> Switch/1
  Relational Operator/1 -> Switch/2
  Divide1/1 -> Relational Operator/2, Output1/1
  Input/1 -> Relational Operator/1

== system lateral_longiitude_distance/Subsystem3/FORWARD_SYSTEM/FORWARD_EMERGENCY_BRAKING_SYSTEM /LESS_THAN_60/Spd_Km_m1 ==
  In1 : Inport
  Constant1 : Constant  Value=1000
  Constant2 : Constant  Value=3600
  Divide : Product  Inputs=*/
  Product : Product
  Out1 : Outport
  wires:
  In1/1 -> Product/1
  Divide/1 -> Out1/1
  Constant2/1 -> Divide/2
  Product/1 -> Divide/1
  Constant1/1 -> Product/2

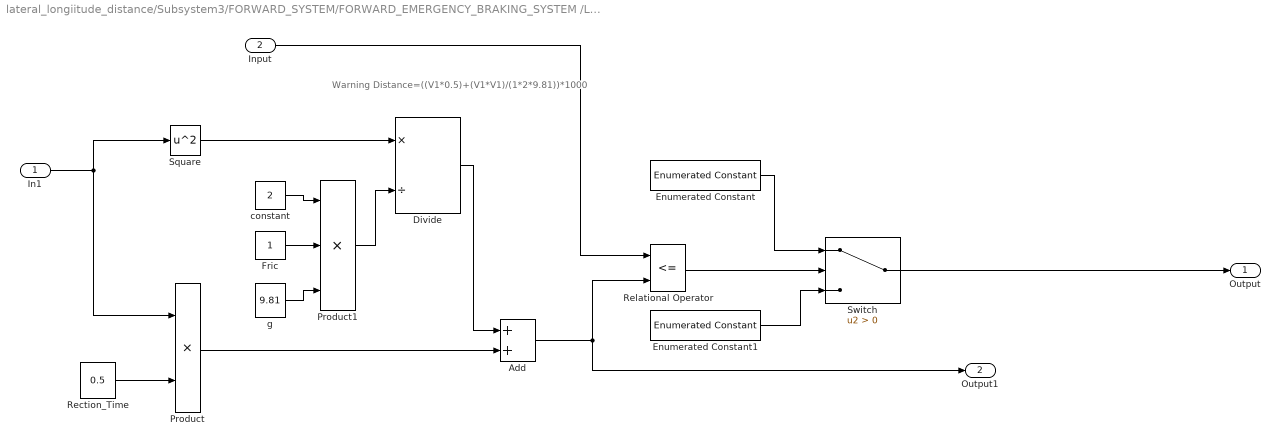
== system lateral_longiitude_distance/Subsystem3/FORWARD_SYSTEM/FORWARD_EMERGENCY_BRAKING_SYSTEM /LESS_THAN_60/W_D ==
  note: Warning Distance=((V1*0.5)+(V1*V1)/(1*2*9.81))*1000
  In1 : Inport
  Input : Inport  Port=2
  Add : Sum
  Divide : Product  Inputs=*/
  Enumerated Constant : simulink/Sources/Enumerated Constant  OutDataTypeStr=Enum: BRAKING_ON_OFF  Value=BRAKING_ON_OFF.FRONT_WARNING_ON  SampleTime=inf
      settings: SourceProductName=Simulink
  Enumerated Constant1 : simulink/Sources/Enumerated Constant  OutDataTypeStr=Enum: BRAKING_ON_OFF  Value=BRAKING_ON_OFF.WARNING_OFF  SampleTime=inf
      settings: SourceProductName=Simulink
  Fric : Constant
  Product : Product
  Product1 : Product  Inputs=3
  "Rection_Time " : Constant  Value=0.5
  Relational Operator : RelationalOperator  Operator=<=  OutDataTypeStr=boolean  RndMeth=Simplest
  Square : Math  Operator=square  SaturateOnIntegerOverflow=on
  Switch : Switch  Criteria=u2 > Threshold
  constant : Constant  Value=2
  g : Constant  Value=9.81
  Output : Outport
  Output1 : Outport  Port=2
  wires:
  Divide/1 -> Add/1
  "Rection_Time "/1 -> Product/2
  In1/1 -> Square/1, Product/1
  Product/1 -> Add/2
  Square/1 -> Divide/1
  g/1 -> Product1/3
  constant/1 -> Product1/1
  Fric/1 -> Product1/2
  Product1/1 -> Divide/2
  Relational Operator/1 -> Switch/2
  Enumerated Constant/1 -> Switch/1
  Enumerated Constant1/1 -> Switch/3
  Input/1 -> Relational Operator/1
  Switch/1 -> Output/1
  Add/1 -> Relational Operator/2, Output1/1

== system lateral_longiitude_distance/Subsystem3/REAR_SYSTEM/REAR_EMERGENCY_BRAKING_SYSTEM /GREATER_THAN_40/B_D ==
  note: Braking Distance=((V1*V1)/(0.7*2*9.81))*1000
  In1 : Inport
  Input : Inport  Port=2
  Divide1 : Product  Inputs=*/
  Enumerated Constant : simulink/Sources/Enumerated Constant  OutDataTypeStr=Enum: BRAKING_ON_OFF  Value=BRAKING_ON_OFF.FRONT_WARNING_ON  SampleTime=inf
      settings: SourceProductName=Simulink
  Enumerated Constant1 : simulink/Sources/Enumerated Constant  OutDataTypeStr=Enum: BRAKING_ON_OFF  Value=BRAKING_ON_OFF.BRAKING_OFF  SampleTime=inf
      settings: SourceProductName=Simulink
  Fric : Constant  Value=0.7
  Product1 : Product  Inputs=3
  Relational Operator : RelationalOperator  Operator=<=  OutDataTypeStr=boolean  RndMeth=Simplest
  Square : Math  Operator=square  SaturateOnIntegerOverflow=on
  Switch : Switch  Criteria=u2 > Threshold
  constant : Constant  Value=2
  g : Constant  Value=9.81
  Output : Outport
  Output1 : Outport  Port=2
  wires:
  Input/1 -> Relational Operator/1
  Divide1/1 -> Output1/1, Relational Operator/2
  Relational Operator/1 -> Switch/2
  Enumerated Constant/1 -> Switch/1
  Enumerated Constant1/1 -> Switch/3
  Switch/1 -> Output/1
  g/1 -> Product1/3
  Product1/1 -> Divide1/2
  Fric/1 -> Product1/1
  constant/1 -> Product1/2
  In1/1 -> Square/1
  Square/1 -> Divide1/1

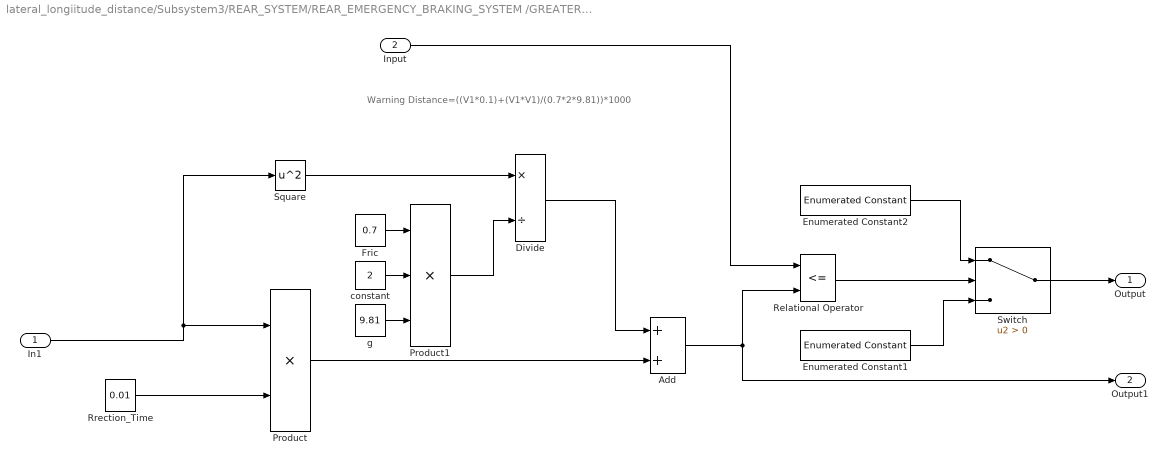
== system lateral_longiitude_distance/Subsystem3/REAR_SYSTEM/REAR_EMERGENCY_BRAKING_SYSTEM /GREATER_THAN_40/W_D ==
  note: Warning Distance=((V1*0.1)+(V1*V1)/(0.7*2*9.81))*1000
  In1 : Inport
  Input : Inport  Port=2
  Add : Sum
  Divide : Product  Inputs=*/
  Enumerated Constant1 : simulink/Sources/Enumerated Constant  OutDataTypeStr=Enum: BRAKING_ON_OFF  Value=BRAKING_ON_OFF.WARNING_OFF  SampleTime=inf
      settings: SourceProductName=Simulink
  Enumerated Constant2 : simulink/Sources/Enumerated Constant  OutDataTypeStr=Enum: BRAKING_ON_OFF  Value=BRAKING_ON_OFF.FRONT_WARNING_ON  SampleTime=inf
      settings: SourceProductName=Simulink
  Fric : Constant  Value=0.7
  Product : Product
  Product1 : Product  Inputs=3
  Relational Operator : RelationalOperator  Operator=<=  OutDataTypeStr=boolean  RndMeth=Simplest
  "Rrection_Time " : Constant  Value=0.01
  Square : Math  Operator=square  SaturateOnIntegerOverflow=on
  Switch : Switch  Criteria=u2 > Threshold
  constant : Constant  Value=2
  g : Constant  Value=9.81
  Output : Outport
  Output1 : Outport  Port=2
  wires:
  Input/1 -> Relational Operator/1
  Add/1 -> Relational Operator/2, Output1/1
  Relational Operator/1 -> Switch/2
  Enumerated Constant2/1 -> Switch/1
  Enumerated Constant1/1 -> Switch/3
  Switch/1 -> Output/1
  g/1 -> Product1/3
  constant/1 -> Product1/2
  Fric/1 -> Product1/1
  Divide/1 -> Add/1
  "Rrection_Time "/1 -> Product/2
  In1/1 -> Product/1, Square/1
  Product/1 -> Add/2
  Square/1 -> Divide/1
  Product1/1 -> Divide/2

== system lateral_longiitude_distance/Subsystem3/REAR_SYSTEM/REAR_EMERGENCY_BRAKING_SYSTEM /LESS_THAN_40/B_D ==
  note: Braking Distance=((V1*V1)/(1*2*9.81))
  In1 : Inport
  Input : Inport  Port=2
  Divide1 : Product  Inputs=*/
  Enumerated Constant : simulink/Sources/Enumerated Constant  OutDataTypeStr=Enum: BRAKING_ON_OFF  Value=BRAKING_ON_OFF.REAR_BRAKING_ON  SampleTime=inf
      settings: SourceProductName=Simulink
  Enumerated Constant1 : simulink/Sources/Enumerated Constant  OutDataTypeStr=Enum: BRAKING_ON_OFF  Value=BRAKING_ON_OFF.BRAKING_OFF  SampleTime=inf
      settings: SourceProductName=Simulink
  Fric : Constant
  Product1 : Product  Inputs=3
  Relational Operator : RelationalOperator  Operator=<=  OutDataTypeStr=boolean  RndMeth=Simplest
  Square : Math  Operator=square  SaturateOnIntegerOverflow=on
  Switch : Switch  Criteria=u2 > Threshold
  constant : Constant  Value=2
  g : Constant  Value=9.81
  Output : Outport
  Output1 : Outport  Port=2
  wires:
  Input/1 -> Relational Operator/1
  Divide1/1 -> Output1/1, Relational Operator/2
  Relational Operator/1 -> Switch/2
  Enumerated Constant/1 -> Switch/1
  Enumerated Constant1/1 -> Switch/3
  Switch/1 -> Output/1
  Product1/1 -> Divide1/2
  g/1 -> Product1/3
  Fric/1 -> Product1/2
  constant/1 -> Product1/1
  Square/1 -> Divide1/1
  In1/1 -> Square/1

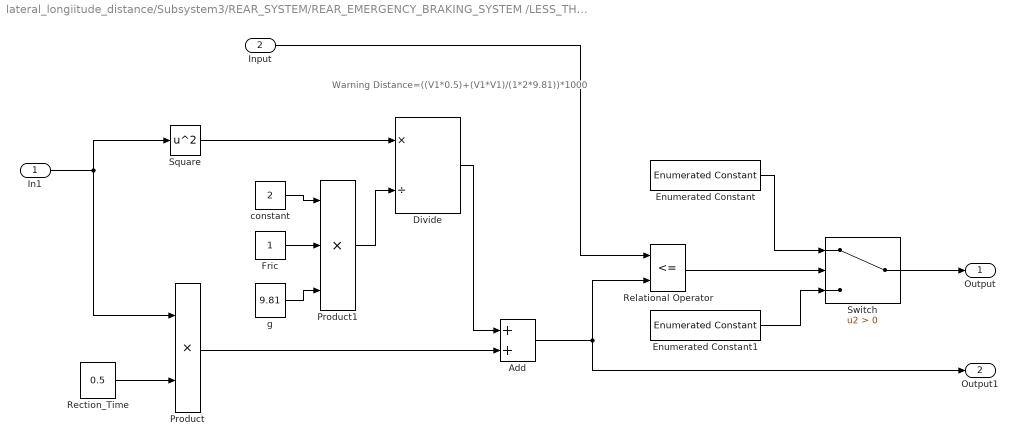
== system lateral_longiitude_distance/Subsystem3/REAR_SYSTEM/REAR_EMERGENCY_BRAKING_SYSTEM /LESS_THAN_40/W_D ==
  note: Warning Distance=((V1*0.5)+(V1*V1)/(1*2*9.81))*1000
  In1 : Inport
  Input : Inport  Port=2
  Add : Sum
  Divide : Product  Inputs=*/
  Enumerated Constant : simulink/Sources/Enumerated Constant  OutDataTypeStr=Enum: BRAKING_ON_OFF  Value=BRAKING_ON_OFF.REAR_WARNING_ON  SampleTime=inf
      settings: SourceProductName=Simulink
  Enumerated Constant1 : simulink/Sources/Enumerated Constant  OutDataTypeStr=Enum: BRAKING_ON_OFF  Value=BRAKING_ON_OFF.WARNING_OFF  SampleTime=inf
      settings: SourceProductName=Simulink
  Fric : Constant
  Product : Product
  Product1 : Product  Inputs=3
  "Rection_Time " : Constant  Value=0.5
  Relational Operator : RelationalOperator  Operator=<=  OutDataTypeStr=boolean  RndMeth=Simplest
  Square : Math  Operator=square  SaturateOnIntegerOverflow=on
  Switch : Switch  Criteria=u2 > Threshold
  constant : Constant  Value=2
  g : Constant  Value=9.81
  Output : Outport
  Output1 : Outport  Port=2
  wires:
  Add/1 -> Output1/1, Relational Operator/2
  Switch/1 -> Output/1
  Input/1 -> Relational Operator/1
  Enumerated Constant1/1 -> Switch/3
  Enumerated Constant/1 -> Switch/1
  Relational Operator/1 -> Switch/2
  Product1/1 -> Divide/2
  Fric/1 -> Product1/2
  constant/1 -> Product1/1
  g/1 -> Product1/3
  Square/1 -> Divide/1
  Product/1 -> Add/2
  In1/1 -> Product/1, Square/1
  "Rection_Time "/1 -> Product/2
  Divide/1 -> Add/1
